simulink model "GammaandTorqueMover"  (R2022b)
settings: Solver=FixedStepAuto  StartTime=0.0  StopTime=10  FixedStep=0.01  RelTol=1e-3
undefined symbols (not defined in the file or in its folder): Kd, Ki, Kp
libraries: mpclib x6, slpidlib x6, simulink x1
(part 1 of 4)
settings Model: Creator=Alireza  LastModifiedBy=Alireza

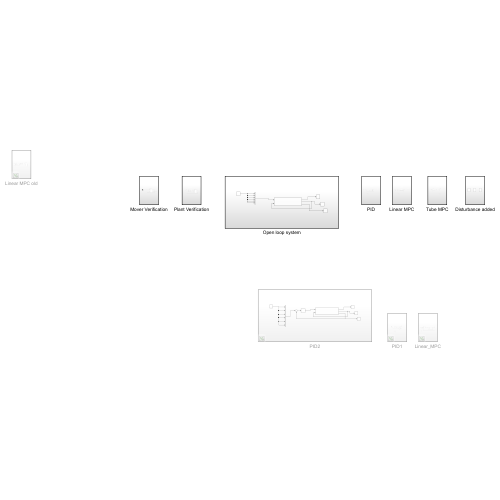
[thumbnail: Simulink's stored preview of the top-level diagram]
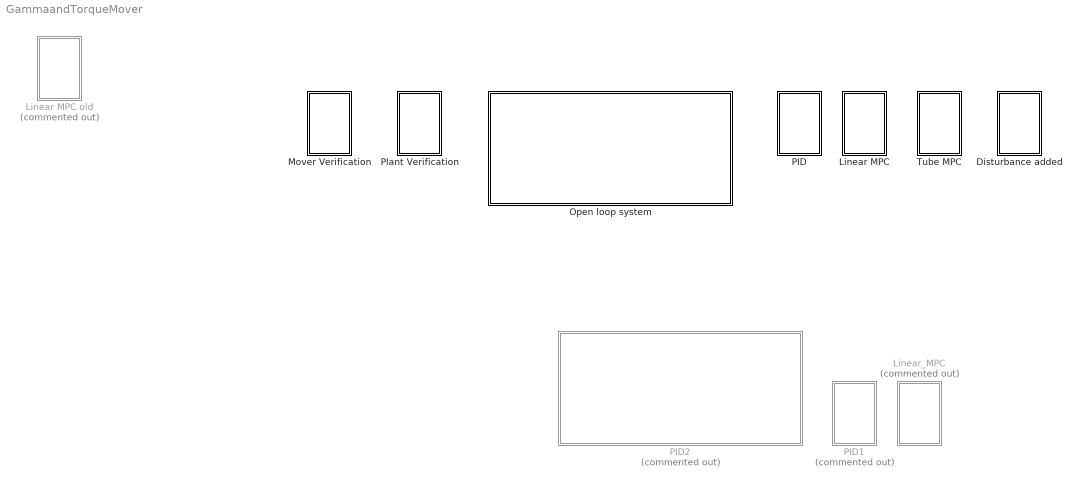
== system GammaandTorqueMover ==
  Disturbance added : Subsystem
  Linear MPC : Subsystem
  Linear MPC old : Subsystem  Commented=on
  Linear_MPC : Subsystem  Commented=on
  Mover Verification : Subsystem
  Open loop system : Subsystem
  PID : Subsystem
  PID1 : Subsystem  Commented=on
  PID2 : Subsystem  Commented=on
  Plant Verification : Subsystem
  Tube MPC : Subsystem

== system GammaandTorqueMover/Disturbance added ==
  Linear MPC plus D : Subsystem
  PID plus D : Subsystem
  Tube MPC plus D : Subsystem

== system GammaandTorqueMover/Linear MPC ==
  note: Gamma and Gamma inverse verified successfully
      | Also the plant works well, but the delay nust have initial condition
  Demux : Demux  Commented=on  Outputs=12
  MLPM Plant1 : Subsystem  Commented=on
  MPC Controller : mpclib/MPC Controller  SCDEnableBlockLinearizationSpecification=on  mpcobj=mpc1  is_multiple=0  enable_value=0  return_u0=off  updateMPCinCallerWorkspace=on  md_inport=off  mv_inport=off  uref_inport=off  return_cost=off  return_mvseq=off  return_qpstatus=off  return_xseq=off  return_state=off  return_ovseq=off  state_inport=off  umin_inport=off  umax_inport=off  ymin_inport=off  ymax_inport=off  cc_inport=off  ywt_inport=off  uwt_inport=off  duwt_inport=off  rhoeps_inport=off  pm_inport=off  MaximumP=13  HorizonChoice=FixedHorizon  n_ts=0.04  n_p=100  n_mv=6  n_md=0  n_ud=0  n_mo=6  n_uo=0  BlockDataType=double  SampleTimeInherited=off  switch_inport=off
  Mux : Mux  Commented=on  Inputs=6
  Mux2 : Mux  Inputs=6
  Scope : Scope
  Scope1 : Scope
  Step : Step  Time=0  SampleTime=0
  Subsystem : Subsystem
  wires:
  Demux/5 -> Mux/3
  Demux/7 -> Mux/4
  Demux/9 -> Mux/5
  Mux/1 -> ?
  Demux/11 -> Mux/6
  Demux/3 -> Mux/2
  Demux/1 -> Mux/1
  ? -> Demux/1  "PID Position and Orientation"
  MPC Controller/1 -> Subsystem/1(Open Loop effort)  "MPC control effort"
  Subsystem/3(Open Loop Position and Orientation) -> MPC Controller/1, Scope1/1  "MPC Position and Orientation"
  Subsystem/1(Open Loop Net Wrench) -> Scope/1  "MPC Net Wrench"
  Subsystem/2(Open Loop states) -> Subsystem/2(position)  "MPC states"
  Mux2/1 -> MPC Controller/2  "MPC Refernce"
  Step/1 -> Mux2/3, Mux2/4, Mux2/6, Mux2/5, Mux2/2, Mux2/1

== system GammaandTorqueMover/Linear MPC old ==
  Demux : Demux  Outputs=6
  Gamma : Subsystem
  MATLAB Function : MATLAB Function  TreatAsAtomicUnit=on
  MPC Controller : mpclib/MPC Controller  SCDEnableBlockLinearizationSpecification=on  is_multiple=0  enable_value=0  return_u0=off  updateMPCinCallerWorkspace=on  md_inport=off  mv_inport=off  uref_inport=off  return_cost=off  return_mvseq=off  return_qpstatus=off  return_xseq=off  return_state=off  return_ovseq=off  state_inport=off  umin_inport=off  umax_inport=off  ymin_inport=off  ymax_inport=off  cc_inport=off  ywt_inport=off  uwt_inport=off  duwt_inport=off  rhoeps_inport=off  pm_inport=off  MaximumP=10  HorizonChoice=FixedHorizon  n_ts=0.1  n_p=10  n_mv=6  n_md=1  n_ud=0  n_mo=6  n_uo=0  BlockDataType=double  SampleTimeInherited=off  switch_inport=off
  Mux2 : Mux  Inputs=6
  PINV : Subsystem
  Scope : Scope
  Scope1 : Scope
  Step : Step  After=0.1  SampleTime=0
  Terminator{,1..3} (4 alike) : Terminator
  Unit Delay1 : UnitDelay  InitialCondition=[0;0;0;0;0;0]  SampleTime=-1  HasFrameUpgradeWarning=on
  wires:
  Unit Delay1/1 -> PINV/1(input)  "effort"
  Demux/3 -> Terminator/1
  Mux2/1 -> MPC Controller/2  "Refernce"
  Gamma/1(net_wrench) -> MATLAB Function/1(u), Scope/1  "Net Wrench"
  Demux/1 -> Gamma/2(x_m), PINV/2(x_m)
  MATLAB Function/2(y) -> Scope1/1  "Position and Orientation"
  Demux/6 -> Terminator3/1
  Step/1 -> Mux2/4, Mux2/5, Mux2/6, Mux2/3, Mux2/2, Mux2/1
  Demux/2 -> Gamma/3(y_m), PINV/3(y_m)
  Demux/5 -> Terminator2/1
  MATLAB Function/1(xdot) -> Demux/1, MATLAB Function/2(x), MPC Controller/1  "states"
  Demux/4 -> Terminator1/1
  PINV/1(Current) -> Gamma/1(input)  "Currents"
  MPC Controller/1 -> Unit Delay1/1  "Control effort"

== system GammaandTorqueMover/Linear_MPC ==
  note: Gamma and Gamma inverse verified successfully
      | Also the plant works well, but the delay nust have initial condition
  Integrator : Integrator  InitialCondition=[0;0;0;0;0;0]  LimitOutput=on  UpperSaturationLimit=5  LowerSaturationLimit=-5
  MLPM Plant : Subsystem
  MPC Controller : mpclib/MPC Controller  SCDEnableBlockLinearizationSpecification=on  is_multiple=0  enable_value=0  return_u0=off  updateMPCinCallerWorkspace=on  md_inport=off  mv_inport=off  uref_inport=off  return_cost=off  return_mvseq=off  return_qpstatus=off  return_xseq=off  return_state=off  return_ovseq=off  state_inport=off  umin_inport=off  umax_inport=off  ymin_inport=off  ymax_inport=off  cc_inport=off  ywt_inport=off  uwt_inport=off  duwt_inport=off  rhoeps_inport=off  pm_inport=off  MaximumP=10  HorizonChoice=FixedHorizon  n_ts=0.01  n_p=10  n_mv=6  n_md=1  n_ud=0  n_mo=6  n_uo=0  BlockDataType=double  SampleTimeInherited=off  switch_inport=off
  Mux2 : Mux  Inputs=6
  Scope : Scope
  Scope1 : Scope
  Step : Step  SampleTime=0
  Unit Delay : UnitDelay  InitialCondition=[0;0;0;0;0;0]  SampleTime=-1  HasFrameUpgradeWarning=on
  wires:
  MLPM Plant/3(MPC Position and Orientation) -> MPC Controller/1, Scope1/1  "MPC Position and Orientation"
  MLPM Plant/1(MPC Net Wrench) -> Scope/1  "MPC Net Wrench"
  Integrator/1 -> MLPM Plant/2(position)
  MPC Controller/1 -> MLPM Plant/1(MPC Control effort)  "MPC Control effort"
  MLPM Plant/2(PID states) -> Integrator/1  "MPC states"
  Mux2/1 -> MPC Controller/2  "MPC Refernce"
  Step/1 -> Mux2/4, Mux2/5, Mux2/6, Mux2/3, Mux2/2, Mux2/1

== system GammaandTorqueMover/Mover Verification ==
  Integrator : Integrator  InitialCondition=[0;0;0;0;0;0;0;0;0;0;0;0]
  MATLAB Function : MATLAB Function  TreatAsAtomicUnit=on
  Mux2 : Mux  Inputs=6
  Scope : Scope
  Scope1 : Scope
  Step : Step  After=0  SampleTime=0
  wires:
  MATLAB Function/2(y) -> Scope1/1  "Mover Response"
  Integrator/1 -> MATLAB Function/2(x)
  Step/1 -> Mux2/4, Mux2/5, Mux2/6, Mux2/3, Mux2/2, Mux2/1
  Mux2/1 -> Scope/1, MATLAB Function/1(u)  "Zero input to Mover"
  MATLAB Function/1(xdot) -> Integrator/1  "Mover Verification states"

== system GammaandTorqueMover/Open loop system ==
  Mux2 : Mux  Inputs=6
  Scope : Scope
  Scope1 : Scope
  Scope2 : Scope
  Step : Step  After=0.1  SampleTime=0
  Subsystem : Subsystem
  wires:
  Step/1 -> Mux2/1, Mux2/2, Mux2/3, Mux2/6, Mux2/5, Mux2/4
  Subsystem/1(Open Loop Net Wrench) -> Scope/1
  Subsystem/3(Open Loop Position and Orientation) -> Scope2/1
  Subsystem/2(Open Loop states) -> Subsystem/2(position), Scope1/1
  Mux2/1 -> Subsystem/1(Open Loop effort)  "Open Loop Refernce"

== system GammaandTorqueMover/PID ==
  note: Gamma and Gamma inverse verified successfully
      | Also the plant works well, but the delay nust have initial condition
  Demux : Demux  Commented=on  Outputs=12
  MLPM Plant1 : Subsystem  Commented=on
  Mux : Mux  Commented=on  Inputs=6
  Mux2 : Mux  Inputs=6
  PID Controller2 : slpidlib/PID Controller  Controller=PID  Form=Parallel  TimeDomain=Continuous-time  UseExternalTs=off  SampleTime=-1  IntegratorMethod=Forward Euler  FilterMethod=Forward Euler  ControllerParametersSource=internal  P=[10000;10000;11000;180;180;200]  I=[4800;4800;50000;400;400;180]  UseKiTs=off  D=[350;350;325;4;4;6.5]  N=100  UseFilter=on  TunerSelectOption=Transfer Function Based (PID Tuner App)  InitialConditionSource=internal  InitialConditionForIntegrator=0  InitialConditionForFilter=0  DifferentiatorICPrevScaledInput=0  ExternalReset=none  TrackingMode=off  Kt=1  LimitOutput=off  SatLimitsSource=internal  UpperSaturationLimit=inf  LowerSaturationLimit=-inf  LinearizeAsGain=on  AntiWindupMode=none  Kb=1  LimitIntegrator=off  UpperIntegratorSaturationLimit=inf  LowerIntegratorSaturationLimit=-inf  POutMin=[]  POutMax=[]  IOutMin=[]  IOutMax=[]  DOutMin=[]  DOutMax=[]  NOutMin=[]  NOutMax=[]  SumOutMin=[]  SumOutMax=[]  SaturationOutMin=[]  SaturationOutMax=[]  PParamMin=[]  PParamMax=[]  IParamMin=[]  IParamMax=[]  DParamMin=[]  DParamMax=[]  NParamMin=[]  NParamMax=[]  KbParamMin=[]  KbParamMax=[]  KtParamMin=[]  KtParamMax=[]  KbOutMin=[]  KbOutMax=[]  KtOutMin=[]  KtOutMax=[]  IntegratorOutMin=[]  IntegratorOutMax=[]  FilterOutMin=[]  FilterOutMax=[]  SumI1OutMin=[]  SumI1OutMax=[]  SumI2OutMin=[]  SumI2OutMax=[]  SumI3OutMin=[]  SumI3OutMax=[]  SumI4OutMin=[]  SumI4OutMax=[]  SumDOutMin=[]  SumDOutMax=[]  DifferentiatorOutMin=[]  DifferentiatorOutMax=[]  FilterDiffOutCoefMin=[]  FilterDiffOutCoefMax=[]  ReciprocalOutMin=[]  ReciprocalOutMax=[]  SumDenOutMin=[]  SumDenOutMax=[]  SumNumOutMin=[]  SumNumOutMax=[]  DivideOutMin=[]  DivideOutMax=[]  UdiffTsProdOutMin=[]  UdiffTsProdOutMax=[]  NTsProdOutMin=[]  NTsProdOutMax=[]  UintegralTsProdOutMin=[]  UintegralTsProdOutMax=[]  UngainTsProdOutMin=[]  UngainTsProdOutMax=[]  ClampingZeroOutDataTypeStr=Inherit: Inherit via back propagation  ClampingZeroOutMin=[]  ClampingZeroOutMax=[]  FilterDenConstantOutDataTypeStr=Inherit: Inherit via back propagation  FilterDenConstantOutMin=[]  FilterDenConstantOutMax=[]  PCopyOutDataTypeStr=Inherit: Inherit via back propagation  PCopyOutMin=[]  PCopyOutMax=[]  NCopyOutDataTypeStr=Inherit: Inherit via back propagation  NCopyOutMin=[]  NCopyOutMax=[]  IntegratorContinuousStateAttributes=''  IntegratorStateMustResolveToSignalObject=off  IntegratorRTWStateStorageClass=Auto  FilterContinuousStateAttributes=''  FilterStateMustResolveToSignalObject=off  FilterRTWStateStorageClass=Auto  ParallelPVariant=InternalParameters  IdealPVariant=Disabled  IVariant=InternalParameters  DVariant=InternalParameters  IntegratorVariant=Continuous  SatVariant=Disabled  AWVariant=Passthrough  PCopyVariant=Disabled  TRVariant=Disabled  FdbkBlocksVariant=Forward  IdealPFdbkVariant=Disabled  SatFdbkVariant=Disabled  DerivativeFilterVariant=ContFilter  NVariant=InternalParameters  NCopyVariant=Disabled  FilterICVariant=InternalICsFilter  IntegratorICVariant=InternalICs  ExternalResetVariant=Disabled  TRSumVariant=Passthrough  SumFdbkVariant=Disabled  SumVariant=Sum_PID  TsampFilterVariant=InternalTs  TsampNgainVariant=Passthrough  TsampIntegralVariant=Passthrough  ExternalSaturationOutDataTypeStr=Inherit: Same as second input
  Scope : Scope
  Scope1 : Scope
  Step : Step  Time=0  SampleTime=0
  Subsystem : Subsystem
  Sum : Sum  Inputs=|+-
  wires:
  Step/1 -> Mux2/1, Mux2/2, Mux2/3, Mux2/6, Mux2/5, Mux2/4
  Mux2/1 -> Sum/1  "PID Refernce"
  Subsystem/2(Open Loop states) -> Subsystem/2(position)  "PID states"
  Subsystem/1(Open Loop Net Wrench) -> Scope/1  "PID Net Wrench"
  Subsystem/3(Open Loop Position and Orientation) -> Sum/2, Scope1/1  "PID Position and Orientation"
  Sum/1 -> PID Controller2/1  "PID error"
  PID Controller2/1 -> Subsystem/1(Open Loop effort)  "PID control effort"
  ? -> Demux/1  "PID Position and Orientation"
  Demux/1 -> Mux/1
  Demux/3 -> Mux/2
  Demux/11 -> Mux/6
  Mux/1 -> ?
  Demux/9 -> Mux/5
  Demux/7 -> Mux/4
  Demux/5 -> Mux/3

== system GammaandTorqueMover/PID1 ==
  note: Gamma and Gamma inverse verified successfully
      | Also the plant works well, but the delay nust have initial condition
  Demux : Demux  Commented=on  Outputs=12
  MLPM Plant1 : Subsystem  Commented=on
  Mux : Mux  Commented=on  Inputs=6
  Mux2 : Mux  Inputs=6
  PID Controller2 : slpidlib/PID Controller  Controller=PID  Form=Parallel  TimeDomain=Continuous-time  UseExternalTs=off  SampleTime=-1  IntegratorMethod=Forward Euler  FilterMethod=Forward Euler  ControllerParametersSource=internal  P=Kp  I=Ki  UseKiTs=off  D=Kd  N=100  UseFilter=on  TunerSelectOption=Transfer Function Based (PID Tuner App)  InitialConditionSource=internal  InitialConditionForIntegrator=0  InitialConditionForFilter=0  DifferentiatorICPrevScaledInput=0  ExternalReset=none  TrackingMode=off  Kt=1  LimitOutput=off  SatLimitsSource=internal  UpperSaturationLimit=inf  LowerSaturationLimit=-inf  LinearizeAsGain=on  AntiWindupMode=none  Kb=1  LimitIntegrator=off  UpperIntegratorSaturationLimit=inf  LowerIntegratorSaturationLimit=-inf  POutMin=[]  POutMax=[]  IOutMin=[]  IOutMax=[]  DOutMin=[]  DOutMax=[]  NOutMin=[]  NOutMax=[]  SumOutMin=[]  SumOutMax=[]  SaturationOutMin=[]  SaturationOutMax=[]  PParamMin=[]  PParamMax=[]  IParamMin=[]  IParamMax=[]  DParamMin=[]  DParamMax=[]  NParamMin=[]  NParamMax=[]  KbParamMin=[]  KbParamMax=[]  KtParamMin=[]  KtParamMax=[]  KbOutMin=[]  KbOutMax=[]  KtOutMin=[]  KtOutMax=[]  IntegratorOutMin=[]  IntegratorOutMax=[]  FilterOutMin=[]  FilterOutMax=[]  SumI1OutMin=[]  SumI1OutMax=[]  SumI2OutMin=[]  SumI2OutMax=[]  SumI3OutMin=[]  SumI3OutMax=[]  SumI4OutMin=[]  SumI4OutMax=[]  SumDOutMin=[]  SumDOutMax=[]  DifferentiatorOutMin=[]  DifferentiatorOutMax=[]  FilterDiffOutCoefMin=[]  FilterDiffOutCoefMax=[]  ReciprocalOutMin=[]  ReciprocalOutMax=[]  SumDenOutMin=[]  SumDenOutMax=[]  SumNumOutMin=[]  SumNumOutMax=[]  DivideOutMin=[]  DivideOutMax=[]  UdiffTsProdOutMin=[]  UdiffTsProdOutMax=[]  NTsProdOutMin=[]  NTsProdOutMax=[]  UintegralTsProdOutMin=[]  UintegralTsProdOutMax=[]  UngainTsProdOutMin=[]  UngainTsProdOutMax=[]  ClampingZeroOutDataTypeStr=Inherit: Inherit via back propagation  ClampingZeroOutMin=[]  ClampingZeroOutMax=[]  FilterDenConstantOutDataTypeStr=Inherit: Inherit via back propagation  FilterDenConstantOutMin=[]  FilterDenConstantOutMax=[]  PCopyOutDataTypeStr=Inherit: Inherit via back propagation  PCopyOutMin=[]  PCopyOutMax=[]  NCopyOutDataTypeStr=Inherit: Inherit via back propagation  NCopyOutMin=[]  NCopyOutMax=[]  IntegratorContinuousStateAttributes=''  IntegratorStateMustResolveToSignalObject=off  IntegratorRTWStateStorageClass=Auto  FilterContinuousStateAttributes=''  FilterStateMustResolveToSignalObject=off  FilterRTWStateStorageClass=Auto  ParallelPVariant=InternalParameters  IdealPVariant=Disabled  IVariant=InternalParameters  DVariant=InternalParameters  IntegratorVariant=Continuous  SatVariant=Disabled  AWVariant=Passthrough  PCopyVariant=Disabled  TRVariant=Disabled  FdbkBlocksVariant=Forward  IdealPFdbkVariant=Disabled  SatFdbkVariant=Disabled  DerivativeFilterVariant=ContFilter  NVariant=InternalParameters  NCopyVariant=Disabled  FilterICVariant=InternalICsFilter  IntegratorICVariant=InternalICs  ExternalResetVariant=Disabled  TRSumVariant=Passthrough  SumFdbkVariant=Disabled  SumVariant=Sum_PID  TsampFilterVariant=InternalTs  TsampNgainVariant=Passthrough  TsampIntegralVariant=Passthrough  ExternalSaturationOutDataTypeStr=Inherit: Same as second input
  Scope : Scope
  Scope1 : Scope
  Step : Step  Time=0  SampleTime=0
  Subsystem : Subsystem
  Sum : Sum  Inputs=|+-
  To Workspace : ToWorkspace  VariableName=y_out  SampleTime=-1
      settings: Save2DSignal=2-D array (concatenate along first dimension)
  wires:
  Demux/5 -> Mux/3
  Demux/7 -> Mux/4
  Demux/9 -> Mux/5
  Mux/1 -> ?
  Demux/11 -> Mux/6
  Demux/3 -> Mux/2
  Demux/1 -> Mux/1
  ? -> Demux/1  "PID Position and Orientation"
  PID Controller2/1 -> Subsystem/1(Open Loop effort)  "PID control effort"
  Sum/1 -> PID Controller2/1  "PID error"
  Subsystem/3(Open Loop Position and Orientation) -> Scope1/1, To Workspace/1, Sum/2  "PID Position and Orientation"
  Subsystem/1(Open Loop Net Wrench) -> Scope/1  "PID Net Wrench"
  Subsystem/2(Open Loop states) -> Subsystem/2(position)  "PID states"
  Mux2/1 -> Sum/1  "PID Refernce"
  Step/1 -> Mux2/4, Mux2/5, Mux2/6, Mux2/3, Mux2/2, Mux2/1

== system GammaandTorqueMover/PID2 ==
  Mux2 : Mux  Inputs=6
  PID Controller : slpidlib/PID Controller  Controller=PID  Form=Parallel  TimeDomain=Continuous-time  UseExternalTs=off  SampleTime=-1  IntegratorMethod=Forward Euler  FilterMethod=Forward Euler  ControllerParametersSource=internal  P=[1;1;1;1;1;1]  I=0  UseKiTs=off  D=0  N=100  UseFilter=on  TunerSelectOption=Transfer Function Based (PID Tuner App)  InitialConditionSource=internal  InitialConditionForIntegrator=0  InitialConditionForFilter=0  DifferentiatorICPrevScaledInput=0  ExternalReset=none  TrackingMode=off  Kt=1  LimitOutput=off  SatLimitsSource=internal  UpperSaturationLimit=inf  LowerSaturationLimit=-inf  LinearizeAsGain=on  AntiWindupMode=none  Kb=1  LimitIntegrator=off  UpperIntegratorSaturationLimit=inf  LowerIntegratorSaturationLimit=-inf  POutMin=[]  POutMax=[]  IOutMin=[]  IOutMax=[]  DOutMin=[]  DOutMax=[]  NOutMin=[]  NOutMax=[]  SumOutMin=[]  SumOutMax=[]  SaturationOutMin=[]  SaturationOutMax=[]  PParamMin=[]  PParamMax=[]  IParamMin=[]  IParamMax=[]  DParamMin=[]  DParamMax=[]  NParamMin=[]  NParamMax=[]  KbParamMin=[]  KbParamMax=[]  KtParamMin=[]  KtParamMax=[]  KbOutMin=[]  KbOutMax=[]  KtOutMin=[]  KtOutMax=[]  IntegratorOutMin=[]  IntegratorOutMax=[]  FilterOutMin=[]  FilterOutMax=[]  SumI1OutMin=[]  SumI1OutMax=[]  SumI2OutMin=[]  SumI2OutMax=[]  SumI3OutMin=[]  SumI3OutMax=[]  SumI4OutMin=[]  SumI4OutMax=[]  SumDOutMin=[]  SumDOutMax=[]  DifferentiatorOutMin=[]  DifferentiatorOutMax=[]  FilterDiffOutCoefMin=[]  FilterDiffOutCoefMax=[]  ReciprocalOutMin=[]  ReciprocalOutMax=[]  SumDenOutMin=[]  SumDenOutMax=[]  SumNumOutMin=[]  SumNumOutMax=[]  DivideOutMin=[]  DivideOutMax=[]  UdiffTsProdOutMin=[]  UdiffTsProdOutMax=[]  NTsProdOutMin=[]  NTsProdOutMax=[]  UintegralTsProdOutMin=[]  UintegralTsProdOutMax=[]  UngainTsProdOutMin=[]  UngainTsProdOutMax=[]  ClampingZeroOutDataTypeStr=Inherit: Inherit via back propagation  ClampingZeroOutMin=[]  ClampingZeroOutMax=[]  FilterDenConstantOutDataTypeStr=Inherit: Inherit via back propagation  FilterDenConstantOutMin=[]  FilterDenConstantOutMax=[]  PCopyOutDataTypeStr=Inherit: Inherit via back propagation  PCopyOutMin=[]  PCopyOutMax=[]  NCopyOutDataTypeStr=Inherit: Inherit via back propagation  NCopyOutMin=[]  NCopyOutMax=[]  IntegratorContinuousStateAttributes=''  IntegratorStateMustResolveToSignalObject=off  IntegratorRTWStateStorageClass=Auto  FilterContinuousStateAttributes=''  FilterStateMustResolveToSignalObject=off  FilterRTWStateStorageClass=Auto  ParallelPVariant=InternalParameters  IdealPVariant=Disabled  IVariant=InternalParameters  DVariant=InternalParameters  IntegratorVariant=Continuous  SatVariant=Disabled  AWVariant=Passthrough  PCopyVariant=Disabled  TRVariant=Disabled  FdbkBlocksVariant=Forward  IdealPFdbkVariant=Disabled  SatFdbkVariant=Disabled  DerivativeFilterVariant=ContFilter  NVariant=InternalParameters  NCopyVariant=Disabled  FilterICVariant=InternalICsFilter  IntegratorICVariant=InternalICs  ExternalResetVariant=Disabled  TRSumVariant=Passthrough  SumFdbkVariant=Disabled  SumVariant=Sum_PID  TsampFilterVariant=InternalTs  TsampNgainVariant=Passthrough  TsampIntegralVariant=Passthrough  ExternalSaturationOutDataTypeStr=Inherit: Same as second input
  Scope : Scope
  Scope1 : Scope
  Scope2 : Scope
  Step : Step  After=0.1  SampleTime=0
  Subsystem : Subsystem
  Sum : Sum  Inputs=|+-
  wires:
  Subsystem/2(Open Loop states) -> Scope1/1, Subsystem/2(position)
  Subsystem/1(Open Loop Net Wrench) -> Scope/1
  Step/1 -> Mux2/2, Mux2/3, Mux2/4, Mux2/5, Mux2/6, Mux2/1
  Mux2/1 -> Sum/1  "Open Loop Refernce"
  Sum/1 -> PID Controller/1
  PID Controller/1 -> Subsystem/1(Open Loop effort)
  Subsystem/3(Open Loop Position and Orientation) -> Scope2/1, Sum/2  "PID Position and Orientation"

== system GammaandTorqueMover/Plant Verification ==
  note: Gamma and Gamma inverse verified successfully
  Gamma : Subsystem
  Integrator : Integrator  InitialCondition=[0;0;0;0;0;0;0;0;0;0;0;0]  LimitOutput=on  UpperSaturationLimit=1  LowerSaturationLimit=-1
  MATLAB Function : MATLAB Function  TreatAsAtomicUnit=on
  Mux2 : Mux  Inputs=6
  PINV : Subsystem
  Scope : Scope
  Scope1 : Scope
  Step : Step  SampleTime=0
  Unit Delay : UnitDelay  InitialCondition=[0;0;0;0;0;0;0;0;0;0;0;0]  SampleTime=-1  HasFrameUpgradeWarning=on
  wires:
  PINV/1(Current) -> Gamma/1(input)  "Currents"
  Step/1 -> Mux2/4, Mux2/5, Mux2/6, Mux2/3, Mux2/2, Mux2/1
  Mux2/1 -> PINV/1(input)  "Verification Input"
  MATLAB Function/2(y) -> Unit Delay/1, Scope1/1  "Position and Orientation"
  Unit Delay/1 -> PINV/2(position), Gamma/2(position)
  Integrator/1 -> MATLAB Function/2(x)
  MATLAB Function/1(xdot) -> Integrator/1  "states"
  Gamma/1(net_wrench) -> MATLAB Function/1(u), Scope/1  "Net Wrench"

== system GammaandTorqueMover/Tube MPC ==
  note: Gamma and Gamma inverse verified successfully
      | Also the plant works well, but the delay nust have initial condition
  Demux : Demux  Commented=on  Outputs=12
  MLPM Plant1 : Subsystem  Commented=on
  MPC Controller : mpclib/MPC Controller  SCDEnableBlockLinearizationSpecification=on  mpcobj=mpc1  is_multiple=0  enable_value=0  return_u0=off  updateMPCinCallerWorkspace=on  md_inport=off  mv_inport=off  uref_inport=off  return_cost=off  return_mvseq=off  return_qpstatus=off  return_xseq=off  return_state=off  return_ovseq=off  state_inport=off  umin_inport=off  umax_inport=off  ymin_inport=off  ymax_inport=off  cc_inport=off  ywt_inport=off  uwt_inport=off  duwt_inport=off  rhoeps_inport=off  pm_inport=off  MaximumP=13  HorizonChoice=FixedHorizon  n_ts=0.04  n_p=100  n_mv=6  n_md=0  n_ud=0  n_mo=6  n_uo=0  BlockDataType=double  SampleTimeInherited=off  switch_inport=off
  Mux : Mux  Commented=on  Inputs=6
  Mux2 : Mux  Inputs=6
  PID Controller1 : slpidlib/PID Controller  Controller=PID  Form=Parallel  TimeDomain=Continuous-time  UseExternalTs=off  SampleTime=-1  IntegratorMethod=Forward Euler  FilterMethod=Forward Euler  ControllerParametersSource=internal  P=[10000;10000;5000;100;100;200]  I=[4800;4800;500;80;80;180]  UseKiTs=off  D=[350;350;100;4;4;6.5]  N=100  UseFilter=on  TunerSelectOption=Transfer Function Based (PID Tuner App)  InitialConditionSource=internal  InitialConditionForIntegrator=0  InitialConditionForFilter=0  DifferentiatorICPrevScaledInput=0  ExternalReset=none  TrackingMode=off  Kt=1  LimitOutput=off  SatLimitsSource=internal  UpperSaturationLimit=inf  LowerSaturationLimit=-inf  LinearizeAsGain=on  AntiWindupMode=none  Kb=1  LimitIntegrator=off  UpperIntegratorSaturationLimit=inf  LowerIntegratorSaturationLimit=-inf  POutMin=[]  POutMax=[]  IOutMin=[]  IOutMax=[]  DOutMin=[]  DOutMax=[]  NOutMin=[]  NOutMax=[]  SumOutMin=[]  SumOutMax=[]  SaturationOutMin=[]  SaturationOutMax=[]  PParamMin=[]  PParamMax=[]  IParamMin=[]  IParamMax=[]  DParamMin=[]  DParamMax=[]  NParamMin=[]  NParamMax=[]  KbParamMin=[]  KbParamMax=[]  KtParamMin=[]  KtParamMax=[]  KbOutMin=[]  KbOutMax=[]  KtOutMin=[]  KtOutMax=[]  IntegratorOutMin=[]  IntegratorOutMax=[]  FilterOutMin=[]  FilterOutMax=[]  SumI1OutMin=[]  SumI1OutMax=[]  SumI2OutMin=[]  SumI2OutMax=[]  SumI3OutMin=[]  SumI3OutMax=[]  SumI4OutMin=[]  SumI4OutMax=[]  SumDOutMin=[]  SumDOutMax=[]  DifferentiatorOutMin=[]  DifferentiatorOutMax=[]  FilterDiffOutCoefMin=[]  FilterDiffOutCoefMax=[]  ReciprocalOutMin=[]  ReciprocalOutMax=[]  SumDenOutMin=[]  SumDenOutMax=[]  SumNumOutMin=[]  SumNumOutMax=[]  DivideOutMin=[]  DivideOutMax=[]  UdiffTsProdOutMin=[]  UdiffTsProdOutMax=[]  NTsProdOutMin=[]  NTsProdOutMax=[]  UintegralTsProdOutMin=[]  UintegralTsProdOutMax=[]  UngainTsProdOutMin=[]  UngainTsProdOutMax=[]  ClampingZeroOutDataTypeStr=Inherit: Inherit via back propagation  ClampingZeroOutMin=[]  ClampingZeroOutMax=[]  FilterDenConstantOutDataTypeStr=Inherit: Inherit via back propagation  FilterDenConstantOutMin=[]  FilterDenConstantOutMax=[]  PCopyOutDataTypeStr=Inherit: Inherit via back propagation  PCopyOutMin=[]  PCopyOutMax=[]  NCopyOutDataTypeStr=Inherit: Inherit via back propagation  NCopyOutMin=[]  NCopyOutMax=[]  IntegratorContinuousStateAttributes=''  IntegratorStateMustResolveToSignalObject=off  IntegratorRTWStateStorageClass=Auto  FilterContinuousStateAttributes=''  FilterStateMustResolveToSignalObject=off  FilterRTWStateStorageClass=Auto  ParallelPVariant=InternalParameters  IdealPVariant=Disabled  IVariant=InternalParameters  DVariant=InternalParameters  IntegratorVariant=Continuous  SatVariant=Disabled  AWVariant=Passthrough  PCopyVariant=Disabled  TRVariant=Disabled  FdbkBlocksVariant=Forward  IdealPFdbkVariant=Disabled  SatFdbkVariant=Disabled  DerivativeFilterVariant=ContFilter  NVariant=InternalParameters  NCopyVariant=Disabled  FilterICVariant=InternalICsFilter  IntegratorICVariant=InternalICs  ExternalResetVariant=Disabled  TRSumVariant=Passthrough  SumFdbkVariant=Disabled  SumVariant=Sum_PID  TsampFilterVariant=InternalTs  TsampNgainVariant=Passthrough  TsampIntegralVariant=Passthrough  ExternalSaturationOutDataTypeStr=Inherit: Same as second input
  Scope : Scope
  Scope1 : Scope
  Step : Step  Time=0  SampleTime=0
  Subsystem : Subsystem
  Sum : Sum  Inputs=|++
  Sum1 : Sum  Inputs=-+|
  wires:
  Step/1 -> Mux2/1, Mux2/2, Mux2/3, Mux2/5, Mux2/6, Mux2/4
  Mux2/1 -> Sum1/2, MPC Controller/2  "Tube MPC Refernce"
  Subsystem/2(Open Loop states) -> Subsystem/2(position)  "Tube MPC states"
  Subsystem/1(Open Loop Net Wrench) -> Scope/1  "Tube MPC Net Wrench"
  Subsystem/3(Open Loop Position and Orientation) -> Scope1/1, MPC Controller/1, Sum1/1  "Tube MPC Position and Orientation"
  MPC Controller/1 -> Sum/1  "Tube MPC_MPC control effort"
  ? -> Demux/1  "PID Position and Orientation"
  Demux/1 -> Mux/1
  Demux/3 -> Mux/2
  Demux/11 -> Mux/6
  Mux/1 -> ?
  Demux/9 -> Mux/5
  Demux/7 -> Mux/4
  Demux/5 -> Mux/3
  PID Controller1/1 -> Sum/2  "Tube MPC_PID control effort"
  Sum/1 -> Subsystem/1(Open Loop effort)  "Tube MPC Control Effort"
  Sum1/1 -> PID Controller1/1

== system GammaandTorqueMover/Disturbance added/Linear MPC plus D ==
  note: Gamma and Gamma inverse verified successfully
      | Also the plant works well, but the delay nust have initial condition
  Demux : Demux  Commented=on  Outputs=12
  MLPM Plant1 : Subsystem  Commented=on
  MPC Controller : mpclib/MPC Controller  SCDEnableBlockLinearizationSpecification=on  mpcobj=mpc1  is_multiple=0  enable_value=0  return_u0=off  updateMPCinCallerWorkspace=on  md_inport=off  mv_inport=off  uref_inport=off  return_cost=off  return_mvseq=off  return_qpstatus=off  return_xseq=off  return_state=off  return_ovseq=off  state_inport=off  umin_inport=off  umax_inport=off  ymin_inport=off  ymax_inport=off  cc_inport=off  ywt_inport=off  uwt_inport=off  duwt_inport=off  rhoeps_inport=off  pm_inport=off  MaximumP=13  HorizonChoice=FixedHorizon  n_ts=0.04  n_p=100  n_mv=6  n_md=0  n_ud=0  n_mo=6  n_uo=0  BlockDataType=double  SampleTimeInherited=off  switch_inport=off
  Mux : Mux  Commented=on  Inputs=6
  Mux2 : Mux  Inputs=6
  Scope : Scope
  Scope1 : Scope
  Step : Step  Time=0  SampleTime=0
  Subsystem : Subsystem
  wires:
  Step/1 -> Mux2/1, Mux2/2, Mux2/5, Mux2/6, Mux2/4, Mux2/3
  Mux2/1 -> MPC Controller/2  "MPC Refernce"
  Subsystem/2(Open Loop states) -> Subsystem/2(position)  "MPC states"
  Subsystem/1(Open Loop Net Wrench) -> Scope/1  "MPC Net Wrench"
  Subsystem/3(Open Loop Position and Orientation) -> Scope1/1, MPC Controller/1  "MPC Position and Orientation"
  MPC Controller/1 -> Subsystem/1(Open Loop effort)  "MPC control effort"
  ? -> Demux/1  "PID Position and Orientation"
  Demux/1 -> Mux/1
  Demux/3 -> Mux/2
  Demux/11 -> Mux/6
  Mux/1 -> ?
  Demux/9 -> Mux/5
  Demux/7 -> Mux/4
  Demux/5 -> Mux/3

== system GammaandTorqueMover/Disturbance added/PID plus D ==
  note: Gamma and Gamma inverse verified successfully
      | Also the plant works well, but the delay nust have initial condition
  Demux : Demux  Commented=on  Outputs=12
  MLPM Plant1 : Subsystem  Commented=on
  Mux : Mux  Commented=on  Inputs=6
  Mux2 : Mux  Inputs=6
  PID Controller2 : slpidlib/PID Controller  Controller=PID  Form=Parallel  TimeDomain=Continuous-time  UseExternalTs=off  SampleTime=-1  IntegratorMethod=Forward Euler  FilterMethod=Forward Euler  ControllerParametersSource=internal  P=[10000;10000;11000;180;180;200]  I=[4800;4800;50000;400;400;180]  UseKiTs=off  D=[350;350;325;4;4;6.5]  N=100  UseFilter=on  TunerSelectOption=Transfer Function Based (PID Tuner App)  InitialConditionSource=internal  InitialConditionForIntegrator=0  InitialConditionForFilter=0  DifferentiatorICPrevScaledInput=0  ExternalReset=none  TrackingMode=off  Kt=1  LimitOutput=off  SatLimitsSource=internal  UpperSaturationLimit=inf  LowerSaturationLimit=-inf  LinearizeAsGain=on  AntiWindupMode=none  Kb=1  LimitIntegrator=off  UpperIntegratorSaturationLimit=inf  LowerIntegratorSaturationLimit=-inf  POutMin=[]  POutMax=[]  IOutMin=[]  IOutMax=[]  DOutMin=[]  DOutMax=[]  NOutMin=[]  NOutMax=[]  SumOutMin=[]  SumOutMax=[]  SaturationOutMin=[]  SaturationOutMax=[]  PParamMin=[]  PParamMax=[]  IParamMin=[]  IParamMax=[]  DParamMin=[]  DParamMax=[]  NParamMin=[]  NParamMax=[]  KbParamMin=[]  KbParamMax=[]  KtParamMin=[]  KtParamMax=[]  KbOutMin=[]  KbOutMax=[]  KtOutMin=[]  KtOutMax=[]  IntegratorOutMin=[]  IntegratorOutMax=[]  FilterOutMin=[]  FilterOutMax=[]  SumI1OutMin=[]  SumI1OutMax=[]  SumI2OutMin=[]  SumI2OutMax=[]  SumI3OutMin=[]  SumI3OutMax=[]  SumI4OutMin=[]  SumI4OutMax=[]  SumDOutMin=[]  SumDOutMax=[]  DifferentiatorOutMin=[]  DifferentiatorOutMax=[]  FilterDiffOutCoefMin=[]  FilterDiffOutCoefMax=[]  ReciprocalOutMin=[]  ReciprocalOutMax=[]  SumDenOutMin=[]  SumDenOutMax=[]  SumNumOutMin=[]  SumNumOutMax=[]  DivideOutMin=[]  DivideOutMax=[]  UdiffTsProdOutMin=[]  UdiffTsProdOutMax=[]  NTsProdOutMin=[]  NTsProdOutMax=[]  UintegralTsProdOutMin=[]  UintegralTsProdOutMax=[]  UngainTsProdOutMin=[]  UngainTsProdOutMax=[]  ClampingZeroOutDataTypeStr=Inherit: Inherit via back propagation  ClampingZeroOutMin=[]  ClampingZeroOutMax=[]  FilterDenConstantOutDataTypeStr=Inherit: Inherit via back propagation  FilterDenConstantOutMin=[]  FilterDenConstantOutMax=[]  PCopyOutDataTypeStr=Inherit: Inherit via back propagation  PCopyOutMin=[]  PCopyOutMax=[]  NCopyOutDataTypeStr=Inherit: Inherit via back propagation  NCopyOutMin=[]  NCopyOutMax=[]  IntegratorContinuousStateAttributes=''  IntegratorStateMustResolveToSignalObject=off  IntegratorRTWStateStorageClass=Auto  FilterContinuousStateAttributes=''  FilterStateMustResolveToSignalObject=off  FilterRTWStateStorageClass=Auto  ParallelPVariant=InternalParameters  IdealPVariant=Disabled  IVariant=InternalParameters  DVariant=InternalParameters  IntegratorVariant=Continuous  SatVariant=Disabled  AWVariant=Passthrough  PCopyVariant=Disabled  TRVariant=Disabled  FdbkBlocksVariant=Forward  IdealPFdbkVariant=Disabled  SatFdbkVariant=Disabled  DerivativeFilterVariant=ContFilter  NVariant=InternalParameters  NCopyVariant=Disabled  FilterICVariant=InternalICsFilter  IntegratorICVariant=InternalICs  ExternalResetVariant=Disabled  TRSumVariant=Passthrough  SumFdbkVariant=Disabled  SumVariant=Sum_PID  TsampFilterVariant=InternalTs  TsampNgainVariant=Passthrough  TsampIntegralVariant=Passthrough  ExternalSaturationOutDataTypeStr=Inherit: Same as second input
  Scope : Scope
  Scope1 : Scope
  Step : Step  Time=0  SampleTime=0
  Subsystem : Subsystem
  Sum : Sum  Inputs=|+-
  wires:
  Demux/5 -> Mux/3
  Demux/7 -> Mux/4
  Demux/9 -> Mux/5
  Mux/1 -> ?
  Demux/11 -> Mux/6
  Demux/3 -> Mux/2
  Demux/1 -> Mux/1
  ? -> Demux/1  "PID Position and Orientation"
  PID Controller2/1 -> Subsystem/1(Open Loop effort)  "PID control effort"
  Sum/1 -> PID Controller2/1  "PID error"
  Subsystem/3(Open Loop Position and Orientation) -> Scope1/1, Sum/2  "PID Position and Orientation"
  Subsystem/1(Open Loop Net Wrench) -> Scope/1  "PID Net Wrench"
  Subsystem/2(Open Loop states) -> Subsystem/2(position)  "PID states"
  Mux2/1 -> Sum/1  "PID Refernce"
  Step/1 -> Mux2/4, Mux2/5, Mux2/6, Mux2/3, Mux2/2, Mux2/1

== system GammaandTorqueMover/Disturbance added/Tube MPC plus D ==
  note: Gamma and Gamma inverse verified successfully
      | Also the plant works well, but the delay nust have initial condition
  Demux : Demux  Commented=on  Outputs=12
  MLPM Plant1 : Subsystem  Commented=on
  MPC Controller : mpclib/MPC Controller  SCDEnableBlockLinearizationSpecification=on  mpcobj=mpc1  is_multiple=0  enable_value=0  return_u0=off  updateMPCinCallerWorkspace=on  md_inport=off  mv_inport=off  uref_inport=off  return_cost=off  return_mvseq=off  return_qpstatus=off  return_xseq=off  return_state=off  return_ovseq=off  state_inport=off  umin_inport=off  umax_inport=off  ymin_inport=off  ymax_inport=off  cc_inport=off  ywt_inport=off  uwt_inport=off  duwt_inport=off  rhoeps_inport=off  pm_inport=off  MaximumP=13  HorizonChoice=FixedHorizon  n_ts=0.04  n_p=100  n_mv=6  n_md=0  n_ud=0  n_mo=6  n_uo=0  BlockDataType=double  SampleTimeInherited=off  switch_inport=off
  Mux : Mux  Commented=on  Inputs=6
  Mux2 : Mux  Inputs=6
  PID Controller1 : slpidlib/PID Controller  Controller=PID  Form=Parallel  TimeDomain=Continuous-time  UseExternalTs=off  SampleTime=-1  IntegratorMethod=Forward Euler  FilterMethod=Forward Euler  ControllerParametersSource=internal  P=[10000;10000;5000;100;100;200]  I=[4800;4800;500;80;80;180]  UseKiTs=off  D=[350;350;100;4;4;6.5]  N=100  UseFilter=on  TunerSelectOption=Transfer Function Based (PID Tuner App)  InitialConditionSource=internal  InitialConditionForIntegrator=0  InitialConditionForFilter=0  DifferentiatorICPrevScaledInput=0  ExternalReset=none  TrackingMode=off  Kt=1  LimitOutput=off  SatLimitsSource=internal  UpperSaturationLimit=inf  LowerSaturationLimit=-inf  LinearizeAsGain=on  AntiWindupMode=none  Kb=1  LimitIntegrator=off  UpperIntegratorSaturationLimit=inf  LowerIntegratorSaturationLimit=-inf  POutMin=[]  POutMax=[]  IOutMin=[]  IOutMax=[]  DOutMin=[]  DOutMax=[]  NOutMin=[]  NOutMax=[]  SumOutMin=[]  SumOutMax=[]  SaturationOutMin=[]  SaturationOutMax=[]  PParamMin=[]  PParamMax=[]  IParamMin=[]  IParamMax=[]  DParamMin=[]  DParamMax=[]  NParamMin=[]  NParamMax=[]  KbParamMin=[]  KbParamMax=[]  KtParamMin=[]  KtParamMax=[]  KbOutMin=[]  KbOutMax=[]  KtOutMin=[]  KtOutMax=[]  IntegratorOutMin=[]  IntegratorOutMax=[]  FilterOutMin=[]  FilterOutMax=[]  SumI1OutMin=[]  SumI1OutMax=[]  SumI2OutMin=[]  SumI2OutMax=[]  SumI3OutMin=[]  SumI3OutMax=[]  SumI4OutMin=[]  SumI4OutMax=[]  SumDOutMin=[]  SumDOutMax=[]  DifferentiatorOutMin=[]  DifferentiatorOutMax=[]  FilterDiffOutCoefMin=[]  FilterDiffOutCoefMax=[]  ReciprocalOutMin=[]  ReciprocalOutMax=[]  SumDenOutMin=[]  SumDenOutMax=[]  SumNumOutMin=[]  SumNumOutMax=[]  DivideOutMin=[]  DivideOutMax=[]  UdiffTsProdOutMin=[]  UdiffTsProdOutMax=[]  NTsProdOutMin=[]  NTsProdOutMax=[]  UintegralTsProdOutMin=[]  UintegralTsProdOutMax=[]  UngainTsProdOutMin=[]  UngainTsProdOutMax=[]  ClampingZeroOutDataTypeStr=Inherit: Inherit via back propagation  ClampingZeroOutMin=[]  ClampingZeroOutMax=[]  FilterDenConstantOutDataTypeStr=Inherit: Inherit via back propagation  FilterDenConstantOutMin=[]  FilterDenConstantOutMax=[]  PCopyOutDataTypeStr=Inherit: Inherit via back propagation  PCopyOutMin=[]  PCopyOutMax=[]  NCopyOutDataTypeStr=Inherit: Inherit via back propagation  NCopyOutMin=[]  NCopyOutMax=[]  IntegratorContinuousStateAttributes=''  IntegratorStateMustResolveToSignalObject=off  IntegratorRTWStateStorageClass=Auto  FilterContinuousStateAttributes=''  FilterStateMustResolveToSignalObject=off  FilterRTWStateStorageClass=Auto  ParallelPVariant=InternalParameters  IdealPVariant=Disabled  IVariant=InternalParameters  DVariant=InternalParameters  IntegratorVariant=Continuous  SatVariant=Disabled  AWVariant=Passthrough  PCopyVariant=Disabled  TRVariant=Disabled  FdbkBlocksVariant=Forward  IdealPFdbkVariant=Disabled  SatFdbkVariant=Disabled  DerivativeFilterVariant=ContFilter  NVariant=InternalParameters  NCopyVariant=Disabled  FilterICVariant=InternalICsFilter  IntegratorICVariant=InternalICs  ExternalResetVariant=Disabled  TRSumVariant=Passthrough  SumFdbkVariant=Disabled  SumVariant=Sum_PID  TsampFilterVariant=InternalTs  TsampNgainVariant=Passthrough  TsampIntegralVariant=Passthrough  ExternalSaturationOutDataTypeStr=Inherit: Same as second input
  Scope : Scope
  Scope1 : Scope
  Step : Step  Time=0  SampleTime=0
  Subsystem : Subsystem
  Sum : Sum  Inputs=|++
  Sum1 : Sum  Inputs=-+|
  wires:
  Sum1/1 -> PID Controller1/1
  Sum/1 -> Subsystem/1(Open Loop effort)  "Tube MPC Control Effort"
  PID Controller1/1 -> Sum/2  "Tube MPC_PID control effort"
  Demux/5 -> Mux/3
  Demux/7 -> Mux/4
  Demux/9 -> Mux/5
  Mux/1 -> ?
  Demux/11 -> Mux/6
  Demux/3 -> Mux/2
  Demux/1 -> Mux/1
  ? -> Demux/1  "PID Position and Orientation"
  MPC Controller/1 -> Sum/1  "Tube MPC_MPC control effort"
  Subsystem/3(Open Loop Position and Orientation) -> Sum1/1, MPC Controller/1, Scope1/1  "Tube MPC Position and Orientation"
  Subsystem/1(Open Loop Net Wrench) -> Scope/1  "Tube MPC Net Wrench"
  Subsystem/2(Open Loop states) -> Subsystem/2(position)  "Tube MPC states"
  Mux2/1 -> MPC Controller/2, Sum1/2  "Tube MPC Refernce"
  Step/1 -> Mux2/4, Mux2/6, Mux2/5, Mux2/3, Mux2/2, Mux2/1

== system GammaandTorqueMover/Linear MPC/MLPM Plant1 ==
  PID Control effort : Inport
  position : Inport  Port=2
  Gamma : Subsystem
  Gravity : Constant  Value=[0;0;-647.2369;0;0;0]
  MATLAB Function : MATLAB Function  TreatAsAtomicUnit=on
  PINV : Subsystem
  Sum1 : Sum  Inputs=++|
  PID Net Wrench : Outport
  PID states : Outport  Port=2
  PID Position and Orientation : Outport  Port=3
  wires:
  MATLAB Function/1(xdot) -> PID states/1  "PID states"
  Gamma/1(net_wrench) -> Sum1/2  "PID Net Wrench"
  position/1 -> MATLAB Function/2(x), Gamma/2(position), PINV/2(position)
  PINV/1(Current) -> Gamma/1(input)  "PID Currents"
  PID Control effort/1 -> PINV/1(input)
  MATLAB Function/2(y) -> PID Position and Orientation/1  "PID Position and Orientation"
  Gravity/1 -> Sum1/1
  Sum1/1 -> PID Net Wrench/1, MATLAB Function/1(u)  "PID Net Wrench"

== system GammaandTorqueMover/Linear MPC/Subsystem ==
  Open Loop effort : Inport
  position : Inport  Port=2
  Gamma : Subsystem
  Integrator : Integrator  InitialCondition=[0;0;0;0;0;0;0;0;0;0;0;0]  LimitOutput=on  UpperSaturationLimit=5  LowerSaturationLimit=-5
  MATLAB Function : MATLAB Function  TreatAsAtomicUnit=on
  PINV : Subsystem
  Open Loop Net Wrench : Outport
  Open Loop states : Outport  Port=2
  Open Loop Position and Orientation : Outport  Port=3
  wires:
  MATLAB Function/1(xdot) -> Integrator/1  "Open Loop states"
  position/1 -> PINV/2(position), Gamma/2(position), MATLAB Function/2(x)
  MATLAB Function/2(y) -> Open Loop Position and Orientation/1  "Open Loop Position and Orientation"
  Open Loop effort/1 -> PINV/1(input)
  PINV/1(Current) -> Gamma/1(input)  "Open Loop Currents"
  Gamma/1(net_wrench) -> MATLAB Function/1(u), Open Loop Net Wrench/1  "Open Loop Wrench"
  Integrator/1 -> Open Loop states/1  "Open Loop states"

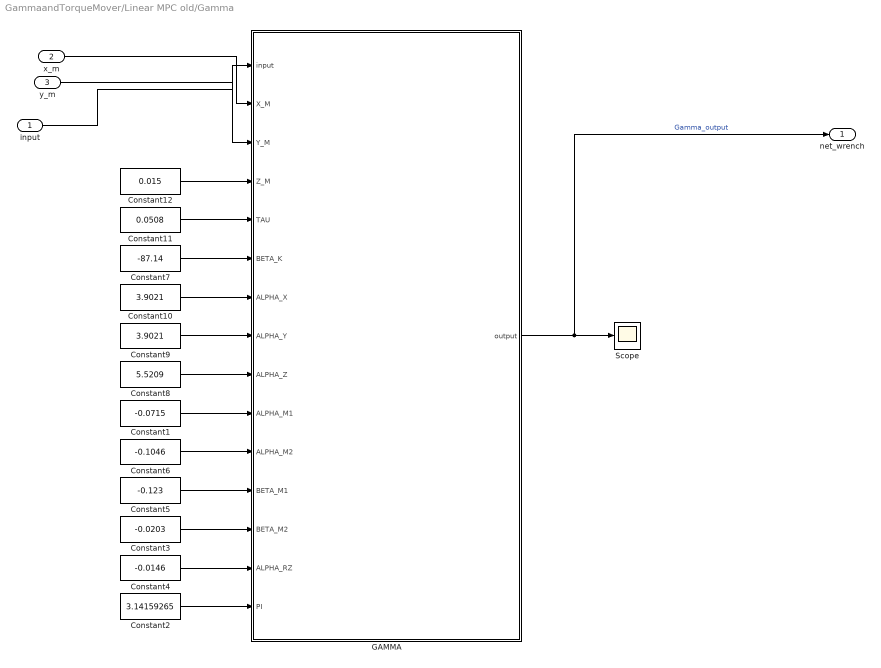
== system GammaandTorqueMover/Linear MPC old/Gamma ==
  input : Inport
  x_m : Inport  Port=2
  y_m : Inport  Port=3
  Constant1 : Constant  Value=-0.0715
  Constant10 : Constant  Value=3.9021
  Constant11 : Constant  Value=0.0508
  Constant12 : Constant  Value=0.015
  Constant2 : Constant  Value=3.14159265
  Constant3 : Constant  Value=-0.0203
  Constant4 : Constant  Value=-0.0146
  Constant5 : Constant  Value=-0.123
  Constant6 : Constant  Value=-0.1046
  Constant7 : Constant  Value=-87.14
  Constant8 : Constant  Value=5.5209
  Constant9 : Constant  Value=3.9021
  GAMMA : MATLAB Function  TreatAsAtomicUnit=on
  Scope : Scope
  net_wrench : Outport
  wires:
  input/1 -> GAMMA/1(input)
  y_m/1 -> GAMMA/3(Y_M)
  x_m/1 -> GAMMA/2(X_M)
  Constant2/1 -> GAMMA/15(PI)
  Constant12/1 -> GAMMA/4(Z_M)
  Constant11/1 -> GAMMA/5(TAU)
  Constant7/1 -> GAMMA/6(BETA_K)
  Constant10/1 -> GAMMA/7(ALPHA_X)
  Constant9/1 -> GAMMA/8(ALPHA_Y)
  Constant8/1 -> GAMMA/9(ALPHA_Z)
  Constant1/1 -> GAMMA/10(ALPHA_M1)
  Constant6/1 -> GAMMA/11(ALPHA_M2)
  Constant5/1 -> GAMMA/12(BETA_M1)
  Constant3/1 -> GAMMA/13(BETA_M2)
  Constant4/1 -> GAMMA/14(ALPHA_RZ)
  GAMMA/1(output) -> net_wrench/1, Scope/1  "Gamma_output"

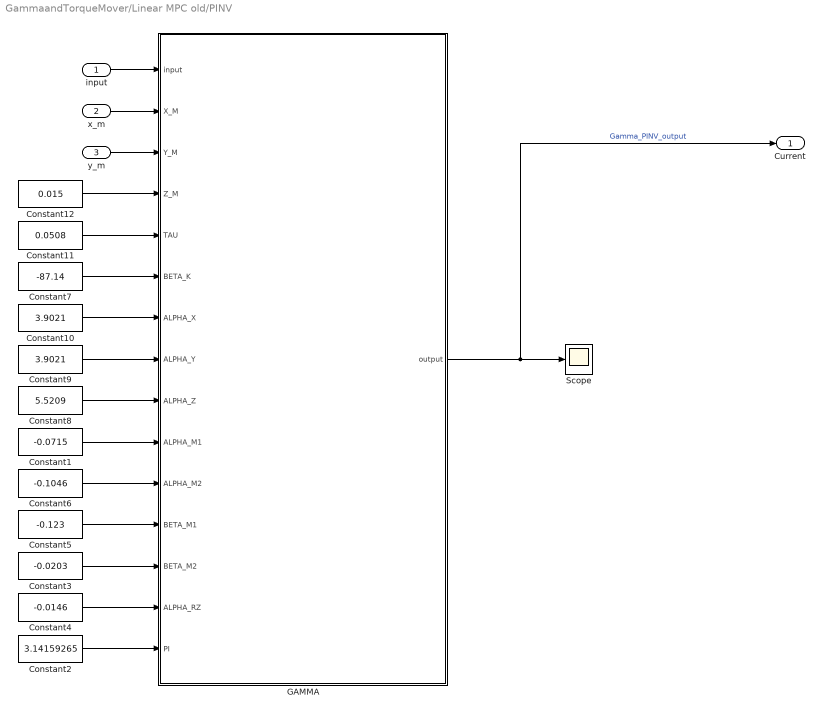
== system GammaandTorqueMover/Linear MPC old/PINV ==
  input : Inport
  x_m : Inport  Port=2
  y_m : Inport  Port=3
  Constant1 : Constant  Value=-0.0715
  Constant10 : Constant  Value=3.9021
  Constant11 : Constant  Value=0.0508
  Constant12 : Constant  Value=0.015
  Constant2 : Constant  Value=3.14159265
  Constant3 : Constant  Value=-0.0203
  Constant4 : Constant  Value=-0.0146
  Constant5 : Constant  Value=-0.123
  Constant6 : Constant  Value=-0.1046
  Constant7 : Constant  Value=-87.14
  Constant8 : Constant  Value=5.5209
  Constant9 : Constant  Value=3.9021
  GAMMA : MATLAB Function  TreatAsAtomicUnit=on
  Scope : Scope
  Current : Outport
  wires:
  Constant4/1 -> GAMMA/14(ALPHA_RZ)
  Constant3/1 -> GAMMA/13(BETA_M2)
  Constant5/1 -> GAMMA/12(BETA_M1)
  Constant6/1 -> GAMMA/11(ALPHA_M2)
  Constant1/1 -> GAMMA/10(ALPHA_M1)
  Constant8/1 -> GAMMA/9(ALPHA_Z)
  Constant9/1 -> GAMMA/8(ALPHA_Y)
  Constant10/1 -> GAMMA/7(ALPHA_X)
  Constant7/1 -> GAMMA/6(BETA_K)
  Constant11/1 -> GAMMA/5(TAU)
  Constant12/1 -> GAMMA/4(Z_M)
  Constant2/1 -> GAMMA/15(PI)
  x_m/1 -> GAMMA/2(X_M)
  y_m/1 -> GAMMA/3(Y_M)
  input/1 -> GAMMA/1(input)
  GAMMA/1(output) -> Current/1, Scope/1  "Gamma_PINV_output"

== system GammaandTorqueMover/Linear_MPC/MLPM Plant ==
  MPC Control effort : Inport
  position : Inport  Port=2
  Gamma : Subsystem
  MATLAB Function : MATLAB Function  TreatAsAtomicUnit=on
  PINV : Subsystem
  MPC Net Wrench : Outport
  PID states : Outport  Port=2
  MPC Position and Orientation : Outport  Port=3
  wires:
  MATLAB Function/2(y) -> MPC Position and Orientation/1  "MPC Position and Orientation"
  MPC Control effort/1 -> PINV/1(input)
  PINV/1(Current) -> Gamma/1(input)  "MPC Currents"
  position/1 -> PINV/2(position), Gamma/2(position), MATLAB Function/2(x)
  Gamma/1(net_wrench) -> MATLAB Function/1(u), MPC Net Wrench/1  "MPC Net Wrench"
  MATLAB Function/1(xdot) -> PID states/1  "MPC states"

== system GammaandTorqueMover/Open loop system/Subsystem ==
  Open Loop effort : Inport
  position : Inport  Port=2
  Gamma : Subsystem
  Integrator : Integrator  InitialCondition=[0;0;0;0;0;0;0;0;0;0;0;0]  LimitOutput=on  UpperSaturationLimit=5  LowerSaturationLimit=-5
  MATLAB Function : MATLAB Function  TreatAsAtomicUnit=on
  PINV : Subsystem
  Open Loop Net Wrench : Outport
  Open Loop states : Outport  Port=2
  Open Loop Position and Orientation : Outport  Port=3
  wires:
  Integrator/1 -> Open Loop states/1  "Open Loop states"
  Gamma/1(net_wrench) -> Open Loop Net Wrench/1, MATLAB Function/1(u)  "Open Loop Wrench"
  PINV/1(Current) -> Gamma/1(input)  "Open Loop Currents"
  Open Loop effort/1 -> PINV/1(input)
  MATLAB Function/2(y) -> Open Loop Position and Orientation/1  "Open Loop Position and Orientation"
  position/1 -> MATLAB Function/2(x), Gamma/2(position), PINV/2(position)
  MATLAB Function/1(xdot) -> Integrator/1  "Open Loop states"

== system GammaandTorqueMover/PID/MLPM Plant1 ==
  PID Control effort : Inport
  position : Inport  Port=2
  Gamma : Subsystem
  Gravity : Constant  Value=[0;0;-647.2369;0;0;0]
  MATLAB Function : MATLAB Function  TreatAsAtomicUnit=on
  PINV : Subsystem
  Sum1 : Sum  Inputs=++|
  PID Net Wrench : Outport
  PID states : Outport  Port=2
  PID Position and Orientation : Outport  Port=3
  wires:
  Sum1/1 -> MATLAB Function/1(u), PID Net Wrench/1  "PID Net Wrench"
  Gravity/1 -> Sum1/1
  MATLAB Function/2(y) -> PID Position and Orientation/1  "PID Position and Orientation"
  PID Control effort/1 -> PINV/1(input)
  PINV/1(Current) -> Gamma/1(input)  "PID Currents"
  position/1 -> PINV/2(position), Gamma/2(position), MATLAB Function/2(x)
  Gamma/1(net_wrench) -> Sum1/2  "PID Net Wrench"
  MATLAB Function/1(xdot) -> PID states/1  "PID states"

== system GammaandTorqueMover/PID/Subsystem ==
  Open Loop effort : Inport
  position : Inport  Port=2
  Gamma : Subsystem
  Integrator : Integrator  InitialCondition=[0;0;0;0;0;0;0;0;0;0;0;0]  LimitOutput=on  UpperSaturationLimit=5  LowerSaturationLimit=-5
  MATLAB Function : MATLAB Function  TreatAsAtomicUnit=on
  PINV : Subsystem
  Open Loop Net Wrench : Outport
  Open Loop states : Outport  Port=2
  Open Loop Position and Orientation : Outport  Port=3
  wires:
  Integrator/1 -> Open Loop states/1  "Open Loop states"
  Gamma/1(net_wrench) -> Open Loop Net Wrench/1, MATLAB Function/1(u)  "Open Loop Wrench"
  PINV/1(Current) -> Gamma/1(input)  "Open Loop Currents"
  Open Loop effort/1 -> PINV/1(input)
  MATLAB Function/2(y) -> Open Loop Position and Orientation/1  "Open Loop Position and Orientation"
  position/1 -> MATLAB Function/2(x), Gamma/2(position), PINV/2(position)
  MATLAB Function/1(xdot) -> Integrator/1  "Open Loop states"

== system GammaandTorqueMover/PID1/MLPM Plant1 ==
  PID Control effort : Inport
  position : Inport  Port=2
  Gamma : Subsystem
  Gravity : Constant  Value=[0;0;-647.2369;0;0;0]
  MATLAB Function : MATLAB Function  TreatAsAtomicUnit=on
  PINV : Subsystem
  Sum1 : Sum  Inputs=++|
  PID Net Wrench : Outport
  PID states : Outport  Port=2
  PID Position and Orientation : Outport  Port=3
  wires:
  MATLAB Function/1(xdot) -> PID states/1  "PID states"
  Gamma/1(net_wrench) -> Sum1/2  "PID Net Wrench"
  position/1 -> MATLAB Function/2(x), Gamma/2(position), PINV/2(position)
  PINV/1(Current) -> Gamma/1(input)  "PID Currents"
  PID Control effort/1 -> PINV/1(input)
  MATLAB Function/2(y) -> PID Position and Orientation/1  "PID Position and Orientation"
  Gravity/1 -> Sum1/1
  Sum1/1 -> PID Net Wrench/1, MATLAB Function/1(u)  "PID Net Wrench"

== system GammaandTorqueMover/PID1/Subsystem ==
  Open Loop effort : Inport
  position : Inport  Port=2
  Gamma : Subsystem
  Integrator : Integrator  InitialCondition=[0;0;0;0;0;0;0;0;0;0;0;0]  LimitOutput=on  UpperSaturationLimit=5  LowerSaturationLimit=-5
  MATLAB Function : MATLAB Function  TreatAsAtomicUnit=on
  PINV : Subsystem
  Saturation : Saturate  UpperLimit=10  LowerLimit=-10
  Open Loop Net Wrench : Outport
  Open Loop states : Outport  Port=2
  Open Loop Position and Orientation : Outport  Port=3
  wires:
  Saturation/1 -> Gamma/1(input)  "Real Currents"
  MATLAB Function/1(xdot) -> Integrator/1  "Open Loop states"
  position/1 -> PINV/2(position), Gamma/2(position), MATLAB Function/2(x)
  MATLAB Function/2(y) -> Open Loop Position and Orientation/1  "Open Loop Position and Orientation"
  Open Loop effort/1 -> PINV/1(input)
  PINV/1(Current) -> Saturation/1  "Open Loop Currents"
  Gamma/1(net_wrench) -> MATLAB Function/1(u), Open Loop Net Wrench/1  "Open Loop Wrench"
  Integrator/1 -> Open Loop states/1  "Open Loop states"

== system GammaandTorqueMover/PID2/Subsystem ==
  Open Loop effort : Inport
  position : Inport  Port=2
  Gamma : Subsystem
  Integrator : Integrator  InitialCondition=[0;0;0;0;0;0;0;0;0;0;0;0]
  MATLAB Function : MATLAB Function  TreatAsAtomicUnit=on
  PINV : Subsystem
  Open Loop Net Wrench : Outport
  Open Loop states : Outport  Port=2
  Open Loop Position and Orientation : Outport  Port=3
  wires:
  MATLAB Function/1(xdot) -> Integrator/1  "Open Loop states"
  position/1 -> PINV/2(position), Gamma/2(position), MATLAB Function/2(x)
  MATLAB Function/2(y) -> Open Loop Position and Orientation/1  "Open Loop Position and Orientation"
  Open Loop effort/1 -> PINV/1(input)
  PINV/1(Current) -> Gamma/1(input)  "Open Loop Currents"
  Gamma/1(net_wrench) -> MATLAB Function/1(u), Open Loop Net Wrench/1  "Open Loop Wrench"
  Integrator/1 -> Open Loop states/1  "Open Loop states"

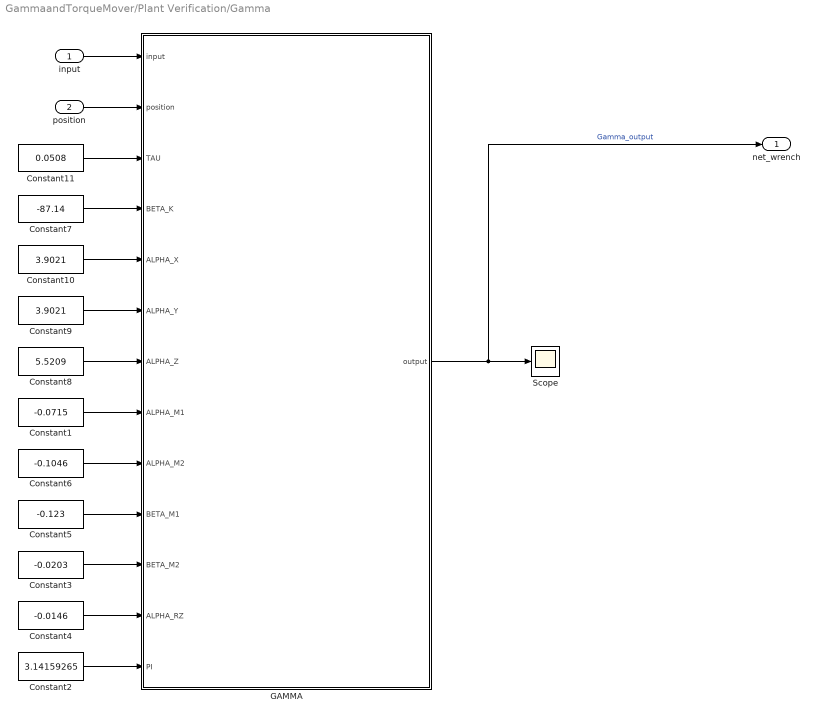
== system GammaandTorqueMover/Plant Verification/Gamma ==
  input : Inport
  position : Inport  Port=2
  Constant1 : Constant  Value=-0.0715
  Constant10 : Constant  Value=3.9021
  Constant11 : Constant  Value=0.0508
  Constant2 : Constant  Value=3.14159265
  Constant3 : Constant  Value=-0.0203
  Constant4 : Constant  Value=-0.0146
  Constant5 : Constant  Value=-0.123
  Constant6 : Constant  Value=-0.1046
  Constant7 : Constant  Value=-87.14
  Constant8 : Constant  Value=5.5209
  Constant9 : Constant  Value=3.9021
  GAMMA : MATLAB Function  TreatAsAtomicUnit=on
  Scope : Scope
  net_wrench : Outport
  wires:
  input/1 -> GAMMA/1(input)
  position/1 -> GAMMA/2(position)
  Constant2/1 -> GAMMA/13(PI)
  Constant11/1 -> GAMMA/3(TAU)
  Constant7/1 -> GAMMA/4(BETA_K)
  Constant10/1 -> GAMMA/5(ALPHA_X)
  Constant9/1 -> GAMMA/6(ALPHA_Y)
  Constant8/1 -> GAMMA/7(ALPHA_Z)
  Constant1/1 -> GAMMA/8(ALPHA_M1)
  Constant6/1 -> GAMMA/9(ALPHA_M2)
  Constant5/1 -> GAMMA/10(BETA_M1)
  Constant3/1 -> GAMMA/11(BETA_M2)
  Constant4/1 -> GAMMA/12(ALPHA_RZ)
  GAMMA/1(output) -> net_wrench/1, Scope/1  "Gamma_output"

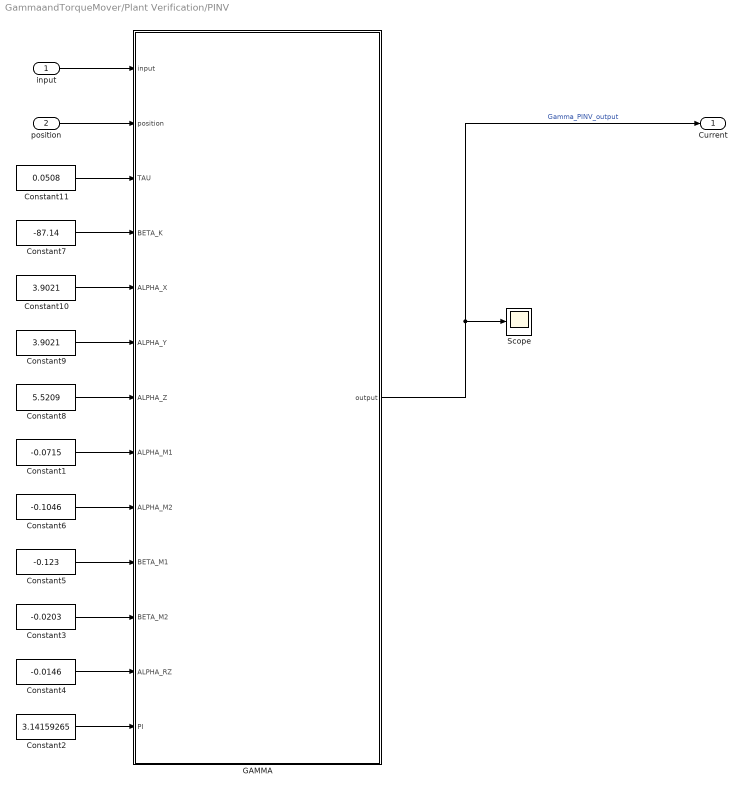
== system GammaandTorqueMover/Plant Verification/PINV ==
  input : Inport
  position : Inport  Port=2
  Constant1 : Constant  Value=-0.0715
  Constant10 : Constant  Value=3.9021
  Constant11 : Constant  Value=0.0508
  Constant2 : Constant  Value=3.14159265
  Constant3 : Constant  Value=-0.0203
  Constant4 : Constant  Value=-0.0146
  Constant5 : Constant  Value=-0.123
  Constant6 : Constant  Value=-0.1046
  Constant7 : Constant  Value=-87.14
  Constant8 : Constant  Value=5.5209
  Constant9 : Constant  Value=3.9021
  GAMMA : MATLAB Function  TreatAsAtomicUnit=on
  Scope : Scope
  Current : Outport
  wires:
  Constant4/1 -> GAMMA/12(ALPHA_RZ)
  Constant3/1 -> GAMMA/11(BETA_M2)
  Constant5/1 -> GAMMA/10(BETA_M1)
  Constant6/1 -> GAMMA/9(ALPHA_M2)
  Constant1/1 -> GAMMA/8(ALPHA_M1)
  Constant8/1 -> GAMMA/7(ALPHA_Z)
  Constant9/1 -> GAMMA/6(ALPHA_Y)
  Constant10/1 -> GAMMA/5(ALPHA_X)
  Constant7/1 -> GAMMA/4(BETA_K)
  Constant11/1 -> GAMMA/3(TAU)
  Constant2/1 -> GAMMA/13(PI)
  position/1 -> GAMMA/2(position)
  input/1 -> GAMMA/1(input)
  GAMMA/1(output) -> Current/1, Scope/1  "Gamma_PINV_output"
